simulink model "MultiUAV_DroneShow"  (R2026a)
settings: Solver=ode1  StopTime=74.3333  FixedStep=Ts_sim  MaxStep=0.01  AbsTol=1e-6
PreLoadFcn:
  | setupParams
values from neighbouring files (symbols this model uses):
  arm_duration = 2    [setupParams.m]
  gnss_deny_mask = false(N_uav, 1)    [setupParams.m]
  gnss_err_gain = sqrt(1 - gnss_err_pole^2)    [setupParams.m]
  gnss_err_pole = exp(-Ts_sim / gnss_err_tau)    [setupParams.m]
  gnss_err_seed = reshape(40000 + (1:(N_uav * 3)), N_uav, 3)    [setupParams.m]
  gps_accuracy_rtk_fix = 0.02    [setupParams.m]
  gps_lock_duration = 2    [setupParams.m]
  gravity = 9.81    [setupParams.m]
  hb_period_ticks = mavlink_hb_interval / Ts_sim    (= 100)    [setupParams.m]
  init_positions = init_positions(pad_of, :)    [planShow.m]    (also in setupParams.m = plan.init_positions)
  Kd_pos = repmat([Kd_xy Kd_xy Kd_z], N_uav, 1)    [setupParams.m]
  Kff_pos = Kd_pos    [setupParams.m]
  Kp_pos = repmat([Kp_xy Kp_xy Kp_z], N_uav, 1)    [setupParams.m]
  land_end_time = plan.land_end_time    [packShowUpload.m]    (also in planShow.m = show_flight_duration + land_duration; setupParams.m)
  land_speed = cfg.land_speed    [planShow.m]
  land_start_time = show_flight_duration    [planShow.m]    (also in setupParams.m = plan.land_start_time)
  land_total_duration = land_duration + land_settle    [planShow.m]    (also in setupParams.m = plan.land_total_duration)
  mav_sys_span = 250    [setupParams.m]
  N_uav = 20    [DroneShowExample.m]    (also in packShowUpload.m = cfg.N_uav; planShow.m = cfg.N_uav; setupParams.m = 10)
  num_waypoints = length(upload_times)    [packShowUpload.m]    (also in setupParams.m = pack.num_waypoints)
  rtcm_data_bytes = 180    [setupParams.m]
  rtcm_interval = 1.0    (= 1)    [setupParams.m]
  rtcm_payload_bytes = 4 * 4 * rtk_n_sat    [setupParams.m]
  rtcm_period_ticks = rtcm_interval / Ts_sim    (= 100)    [setupParams.m]
  rtk_amb_l1_base = 1000000 + mod(97 * (1:rtk_n_sat)', 1009)    [setupParams.m]
  rtk_amb_l1_rover = rtk_amb_l1_base + rtk_amb_l1    [setupParams.m]
  rtk_amb_l2_base = 1000000 + mod(89 * (1:rtk_n_sat)', 1009)    [setupParams.m]
  rtk_amb_l2_rover = rtk_amb_l2_base + rtk_amb_l2    [setupParams.m]
  rtk_base_lla = [42.3601, -71.0589, 10]    [setupParams.m]
  rtk_deny_mask = false(N_uav, 1)    [setupParams.m]
  rtk_f1 = 1575.42e6    (= 1575420000)    [setupParams.m]
  rtk_f2 = 1227.60e6    (= 1227600000)    [setupParams.m]
  rtk_fall_slew = -gps_accuracy_standard / reconverge_time    (= -0.3)    [setupParams.m]
  rtk_fix_thresh_l1 = 0.30    (= 0.3)    [setupParams.m]
  rtk_fix_thresh_wl = 0.25    [setupParams.m]
  rtk_inject_enable = double(~skip_preflight | rtk_deny_mask(:)')    [setupParams.m]
  rtk_lambda1 = rtk_c / rtk_f1    (= 0.190293672798)    [setupParams.m]
  rtk_lambda2 = rtk_c / rtk_f2    (= 0.244210213425)    [setupParams.m]
  rtk_lambda_wl = rtk_c / (rtk_f1 - rtk_f2)    (= 0.861918400322)    [setupParams.m]
  rtk_lock_dwell = 2.0    (= 2)    [setupParams.m]
  rtk_los = [cosd(rtk_el) .* sind(rtk_az), cosd(rtk_el) .* cosd(rtk_az), sind(rtk_el)]    [setupParams.m]
  rtk_mean_clk = zeros(2, 1)    [setupParams.m]
  rtk_mean_obs = zeros(2, rtk_n_sat)    [setupParams.m]
  rtk_n_sat = numel(rtk_az)    [setupParams.m]
  rtk_rough_range = pseudoranges(rtk_base_lla, rtk_sat_pos, 'RangeAccuracy', 0)    [setupParams.m]
  rtk_sat_pos = rtk_sat_pos_all(rtk_vis, :)    [setupParams.m]
  rtk_seedm_clk = 9101 + 8 * rtk_n_sat + (0:1)'    [setupParams.m]
  rtk_seedm_l1 = rtk_seedm_p2 + 2 * rtk_n_sat    [setupParams.m]
  rtk_seedm_l2 = rtk_seedm_l1 + 2 * rtk_n_sat    [setupParams.m]
  rtk_seedm_p1 = 9101 + reshape(0:2 * rtk_n_sat - 1, 2, rtk_n_sat)    [setupParams.m]
  rtk_seedm_p2 = rtk_seedm_p1 + 2 * rtk_n_sat    [setupParams.m]
  rtk_sigma_bp = [0, rtk_timeout, rtk_float_timeout]    [setupParams.m]
  rtk_sigma_table = sqrt(max(0, rtk_sigma_tiers.^2 - gps_accuracy_rtk_fix^2))    [setupParams.m]
  rtk_sigma_unfixed = 0.75    [setupParams.m]
  rtk_slip_thresh_l1 = 0.02    [setupParams.m]
  rtk_slip_thresh_wl = 0.10    (= 0.1)    [setupParams.m]
  rtk_status_l1 = 1    [setupParams.m]
  rtk_status_unfixed = 3    [setupParams.m]
  rtk_timeout = 2.5    [setupParams.m]
  rtk_var_clk = rtk_clock_sigma^2 * ones(2, 1)    [setupParams.m]
  rtk_var_l = [rtk_sigma_phase_base^2; rtk_sigma_phase_rover^2] * ones(1, rtk_n_sat)    [setupParams.m]
  rtk_var_p = [rtk_sigma_code_base^2;  rtk_sigma_code_rover^2 ] * ones(1, rtk_n_sat)    [setupParams.m]
  skip_preflight = traj_source == 1    [DroneShowExample.m]    (also in setupParams.m = false)
  st_period_ticks = mavlink_st_interval / Ts_sim    (= 100)    [setupParams.m]
  st_phase_ticks = st_period_ticks / 2    (= 50)    [setupParams.m]
  telemetry_tx_enable = double(~skip_preflight)    [setupParams.m]
  traj_upload_flat = zeros(N_uav*num_waypoints, 7)    [packShowUpload.m]    (also in setupParams.m = pack.traj_upload_flat)
  Ts_sim = cfg.Ts_sim    [packShowUpload.m]    (also in setupParams.m = 0.01)
  uav_loss_seed = 31000 + (1:N_uav)    [setupParams.m]
  uav_mass = 0.1    [setupParams.m]
  upload_duration = (total_packets + N_uav) * Ts_sim * 1.2    [packShowUpload.m]    (also in setupParams.m = pack.upload_duration)
  upload_rate_vec = [1 ./ upload_dt; 1 / upload_dt(end)]    [packShowUpload.m]    (also in setupParams.m = pack.upload_rate_vec)
  upload_request = traj_source == 2    [DroneShowExample.m]
undefined symbols (not defined in the file or in its folder): abort_request, DiscIntNeverNeededParam, doppler, loss_seed, packet_loss_rate, Payload, SystemID, uav_loss_rate
libraries: uavmavlinklib x22, hdlsllib x16, dspsigops x8, simulink x7, matrix_library x4, commchan3 x2, etargetslib x1, uavalgslib x1, sensorinslib x1, slpidlib x1, dspmathops x1, commrandsrc3 x1
(part 4 of 4)

== matlab function MultiUAV_DroneShow/RTKBase/ObservableSource/Simulated/ObservableGen/Observables ==
  settings: updateMethod=DISCRETE  sampleTime=rtcm_interval
  data: Baseline input; P1 output; Clock input; NoiseP1 input; NoiseP2 input; NoiseL1 input; NoiseL2 input; P2 output; L1 output; L2 output; rtk_base_lla parameter; rtk_sat_pos parameter; rtk_lambda1 parameter; rtk_lambda2 parameter; rtk_amb_l1_base parameter; rtk_amb_l2_base parameter; rtk_amb_l1_rover parameter; rtk_amb_l2_rover parameter
function [P1, P2, L1, L2] = rtkObservables(Baseline, Clock, NoiseP1, NoiseP2, NoiseL1, NoiseL2, rtk_base_lla, rtk_sat_pos, rtk_lambda1, rtk_lambda2, rtk_amb_l1_base, rtk_amb_l2_base, rtk_amb_l1_rover, rtk_amb_l2_rover)
%rtkObservables - what the two receivers measure, UNDIFFERENCED, built from the shipped GNSS functions.
%
% Each output is 2-by-nSat: the BASE row first, then the ROVER row. This is the RTK engine's
% interface, and it is undifferenced on purpose.
%
% WHY UNDIFFERENCED. This block used to emit the between-receiver single difference, which
% made "there are exactly two receivers, and here is how they pair up" an assumption baked
% into the generator. A real base station and a real rover each report their own raw code and
% phase and nothing else; the pairing is the ENGINE's job. Emitting the raw rows instead means
% simulated and measured observables enter the same cascade by the same door -- swap this block
% for a source of real measurements and RTKEngine does not change, which is the point of the
% ObservableSource variant this sits inside. checkRTKEngine arm 15 measures the swap's only
% numerical cost.
%
% Nothing is shared between the two rows except the range's satellite-side content -- the
% satellite clock bias and the Earth-rotation correction that pseudoranges applies -- and that
% content is exactly what the engine's rover-minus-base differencing removes. Each receiver
% gets its OWN clock, its OWN phase counter and its OWN noise amplitude.
%
% Clock is 2-by-1, one draw per receiver at rtk_clock_sigma each. It used to be a single
% pre-differenced scalar, which meant the quantity the cascade exists to cancel was handed to
% it ready-made; now the engine forms it, so arm 1 tests the cascade instead of testing this
% block. It is added identically to all satellites, because that is what makes it cancellable
% -- a per-satellite random term here would not be a clock, it would be undeclared noise that
% no differencing can reach.
%
% NoiseP1..NoiseL2 are 2-by-nSat, base row then rover row, from one Random Number block each.
% The rows carry DIFFERENT amplitudes: rtk_var_p is [0.15^2; 0.30^2] because a survey receiver
% on a pillar with a choke-ring antenna is not a patch antenna bolted to an airframe. The split
% cost no extra blocks -- the Random Number block takes its output dimensions from its
% parameters, so making them 2-by-nSat was enough.
%
% THE PHASE COUNTERS. rtk_amb_l1_base/_rover are the two receivers' own accumulated cycle
% counts, ~1e6 cycles, which puts the raw phase observable at 2.35e7 m -- the magnitude a
% RINEX L1 record has. Their absolute values carry no information; only the difference does,
% and by construction rover minus base is exactly rtk_amb_l1, the ambiguity the engine
% resolves and the tests assert on. Two consequences worth naming:
%   - The differencing is EXACT, not merely accurate. Base and rover agree to a part in 6774,
%     and two doubles within a factor of two of each other subtract with no rounding at all
%     (Sterbenz). What arm 15 measures is the cost of REPRESENTING a raw observable -- adding a
%     900 m clock and centimetres of noise to a 2.35e7 m range, then getting the difference back
%     out: 8.8e-9 m, which is 2.4x eps at that magnitude and 4.0e-6 of the phase noise.
%   - These rows cannot be transmitted as they stand. A SINGLE resolves 2.000 m at 2.35e7 m,
%     so the RTCM payload (rtcm_payload_bytes) carries phase-range RESIDUALS -- observable
%     minus an approximate range -- exactly as a real MSM message does.
%
% WHAT THE RANGE IS. Not a geometric distance: pseudoranges also applies the satellite clock
% bias and the Earth-rotation (Sagnac) correction, which across this constellation run from
% -24.3 m to +20.0 m per satellite. Each is a property of the satellite and the epoch rather
% than of the receiver, so each cancels in the engine's base-rover difference. checkRTKEngine
% arm 12 measures that instead of trusting it, because an uncancelled term would be a
% metre-class satellite-dependent bias, would be indistinguishable from multipath, would be
% absorbed into the integer ambiguities, and would then be reported with a confident centimetre
% sigma. Measured: 24.3 m cancels by a factor of 26246, exactly to zero at zero baseline, and
% leaving 1 m of one satellite's term uncancelled instead costs 0.445 m of position.
%
% What does NOT cancel, and is meant not to: base and rover receive the same signal at transit
% times differing by |b|/c, so the satellite has moved between the two receptions. Arm 6
% decomposes that against the second-order geometric term the old -rtk_los*Baseline form
% dropped:
%
%       |b|      geometric     transit       total
%      62 m       0.087 mm    0.359 mm    0.438 mm
%     200 m       0.901 mm    1.159 mm    1.975 mm
%     500 m       5.630 mm    2.897 mm    7.998 mm
%
% The transit term is LINEAR in the baseline where the geometric term is quadratic, so it
% dominates at show scale -- 4x the geometric term at 62 m -- and a single -los*b product has
% only one satellite position in it and cannot express it at any order.
%
% RangeAccuracy is 0 deliberately. This block supplies the GEOMETRY; every noise term arrives
% on an input port from a Random Number block, seeded per receiver per satellite from
% setupParams. Letting pseudoranges add its own noise would hide an unseeded, unlogged random
% stream inside a MATLAB Function block and make the observables irreproducible.
%#codegen

% Rover geodetic position. The base station sits at the local ENU origin, so the incoming
% Baseline IS the rover's ENU offset from it.
llaRover = enu2lla(Baseline(:)', rtk_base_lla, 'ellipsoid');

pBase  = pseudoranges(rtk_base_lla, rtk_sat_pos, 'RangeAccuracy', 0);
pRover = pseudoranges(llaRover,     rtk_sat_pos, 'RangeAccuracy', 0);

% Base row then rover row, and that order is load-bearing: the engine forms row 2 minus row 1,
% so transposing these two lines would return the negative of the baseline with the base
% clock left in -- and the cascade would still resolve integers around it, just to the wrong
% answer. tests/rtkEngineHarness checks the shape for the same reason.
rho = [pBase(:)'; pRover(:)'];

% One clock per receiver, spread across all satellites.
clk = [Clock(1) * ones(1, numel(pBase)); Clock(2) * ones(1, numel(pBase))];

ambL1 = [rtk_amb_l1_base(:)'; rtk_amb_l1_rover(:)'];
ambL2 = [rtk_amb_l2_base(:)'; rtk_amb_l2_rover(:)'];

P1 = rho + clk + NoiseP1;
P2 = rho + clk + NoiseP2;
L1 = rho + clk + rtk_lambda1 * ambL1 + NoiseL1;
L2 = rho + clk + rtk_lambda2 * ambL2 + NoiseL2;
end

== stateflow chart MultiUAV_DroneShow/RtkGate ==
  settings: updateMethod=DISCRETE  sampleTime=Ts_sim
  state NOT_READY
    en: RtkReady = false;
  state PENDING
    % Status has just claimed a fix. Hold it for rtk_lock_dwell before believing it:
    % the cascade re-validates its held integer set every epoch and un-latches on
    % failure, so an instantaneous test could release the show on an epoch that
    % regresses on the next tick. after() counts from THIS entry, which is why the
    % wait needs its own state.
    en: RtkReady = false;
  state READY
    en: RtkReady = true;
  (default) -> NOT_READY
  READY -> NOT_READY : [RtkStatus ~= rtk_status_l1]
  NOT_READY -> PENDING : [RtkStatus == rtk_status_l1]
  PENDING -> NOT_READY [order 2] : [RtkStatus ~= rtk_status_l1]
  PENDING -> READY [order 1] : [after(rtk_lock_dwell, sec)]
  data: RtkStatus input double; RtkReady output boolean; rtk_lock_dwell parameter double; rtk_status_l1 parameter double

== stateflow chart MultiUAV_DroneShow/BaseStation/MissionProtocol/UploadIndexerBlk/UploadIndexerChart ==
  state IDLE
    entry:
    mode = uint8(0); mc_target = uint16(0); item_target = uint16(0);
    item_seq = uint16(0); lin_idx = uint32(1);
    count_cursor = uint32(0); item_cursor = uint32(0);
    repair_drone = uint32(1); repair_seq = uint16(0);
    stall = uint32(0); repair_done = false; give_up = false;
  state COUNT_PHASE
    during:
    mode = uint8(1);
    mc_target = uint16(count_cursor + 1);
    count_cursor = count_cursor + uint32(1);
    item_target = uint16(0);
    item_seq = uint16(0);
    lin_idx = uint32(1);
  state ITEM_PHASE
    during:
    mode = uint8(2);
    drone_idx = idivide(item_cursor, num_waypoints, 'floor');
    wp_idx = item_cursor - drone_idx*num_waypoints;
    item_target = uint16(drone_idx + 1);
    item_seq = uint16(wp_idx);
    lin_idx = item_cursor + uint32(1);
    item_cursor = item_cursor + uint32(1);
    mc_target = uint16(0);
  state REPAIR
    entry:
    % Gap repair: retransmit only the waypoints a drone reports missing.
    repair_done = false; stall = uint32(0);
    mode = uint8(2); mc_target = uint16(0);
    item_target = uint16(repair_drone); item_seq = repair_seq;
    lin_idx = (repair_drone - uint32(1))*num_waypoints + uint32(repair_seq) + uint32(1);
    during:
    % MISSION_REQUEST_INT names the first waypoint this drone still lacks.
    % seq >= num_waypoints means it has them all, so move to the next drone.
    if req_valid && req_ts == uint16(repair_drone)
    stall = uint32(0);
    if req_seq >= uint16(num_waypoints)
    if repair_drone >= N_uav
    repair_done = true;
    else
    repair_drone = repair_drone + uint32(1);
    repair_seq = uint16(0);
    end
    else
    repair_seq = req_seq;
    end
    else
    % No reply: the item or the request was lost, so resend unchanged.
    stall = stall + uint32(1);
    end
    mode = uint8(2); mc_target = uint16(0);
    item_target = uint16(repair_drone); item_seq = repair_seq;
    lin_idx = (repair_drone - uint32(1))*num_waypoints + uint32(repair_seq) + uint32(1);
  state DONE
    entry:
    mode = uint8(0);
    mc_target = uint16(0);
    item_target = uint16(0);
    item_seq = uint16(0);
    lin_idx = uint32(1);
  state GIVE_UP
    entry:
    mode = uint8(0);
    mc_target = uint16(0);
    item_target = uint16(0);
    item_seq = uint16(0);
    lin_idx = uint32(1);
    give_up = true;
  (default) -> IDLE
  GIVE_UP -> IDLE : [~UploadEnable]
  DONE -> IDLE : [~UploadEnable]
  IDLE -> COUNT_PHASE : [Phase == uint8(1) && UploadEnable && count_cursor < N_uav]
  REPAIR -> IDLE [order 1] : [~UploadEnable]
  ITEM_PHASE -> IDLE [order 1] : [~UploadEnable]
  COUNT_PHASE -> IDLE [order 1] : [~UploadEnable]
  COUNT_PHASE -> ITEM_PHASE [order 2] : [count_cursor >= N_uav]
  ITEM_PHASE -> REPAIR [order 2] : [item_cursor >= N_uav * num_waypoints]
  REPAIR -> DONE [order 2] : [repair_done]
  REPAIR -> GIVE_UP [order 3] : [stall > repair_stall_limit]
  data: Phase input uint8 size=1; UploadEnable input boolean size=1; N_uav input uint32 size=1; num_waypoints input uint32 size=1; mode output uint8 size=1; mc_target output uint16 size=1; item_target output uint16 size=1; item_seq output uint16 size=1; lin_idx output uint32 size=1; count_cursor local uint32 size=1; item_cursor local uint32 size=1; drone_idx local uint32 size=1; wp_idx local uint32 size=1; req_valid input boolean size=[1 1]; req_ts input uint16 size=[1 1]; req_seq input uint16 size=[1 1]; give_up output boolean; repair_drone local uint32; repair_seq local uint16; stall local uint32 size=[1 1]; repair_done local boolean size=[1 1]; repair_stall_limit parameter uint32 size=[1 1]
